simulink model "Warmup"  (R2012b)
settings: Solver=ode1  StartTime=0.0  StopTime=inf  FixedStep=0.001  RelTol=1e-3
PreLoadFcn:
  | prompt = {'Stimulation amplitude [mA]:','Number of pulses:'};
  | dlg_title = 'Warmup Settings';
  | def = {'50','20'};
  | answer = inputdlg(prompt,dlg_title,1,def);
  | amp = str2num(answer{1});
  | np = 1:str2num(answer{2});
  | clear prompt dlg_title def answer
undefined symbols (not defined in the file): HIL, LCconv
libraries: quarc_library x3, simulink x2, ScienceStimHasomed_Lib x1
settings Model: SimulationMode=external  ExtModeTrigDuration=5000000  Creator=LabUser  LastModifiedBy=LabUser
settings SolverCC: PositivePriorityOrder=on
settings DataIOCC: LimitDataPoints=off
settings DebuggingCC: SolverPrmCheckMsg=none
settings RTWCC: SystemTargetFile=quarc_win64.tlc  TemplateMakefile=quarc_default_tmf  Description=QUARC Win64 Target  ProcessScript=quarc_win64_make_rtw_hook
settings RTWCC: CustomLibrary=|
  | sciencemode.obj
  | serial_windows.obj
settings STFCustomTargetCC: TargetPreCompLibLocation=C:\PROGRA~3\QUARC\lib\2012b\win64\release  CodeReplacementLibrary=ANSI_C  GeneratePreprocessorConditionals=Disable all  CombineOutputUpdateFcns=on  GRTInterface=off  SystemTargetFile=quarc_win64.tlc
settings GRTTargetCC: TargetPreCompLibLocation=C:\PROGRA~3\QUARC\lib\2012b\win64\release  ParMdlRefBuildCompliant=off  CompOptLevelCompliant=off  ConcurrentExecutionCompliant=off  MatFileLogging=off  ExtMode=on  ExtModeMexFile=quarc_comm

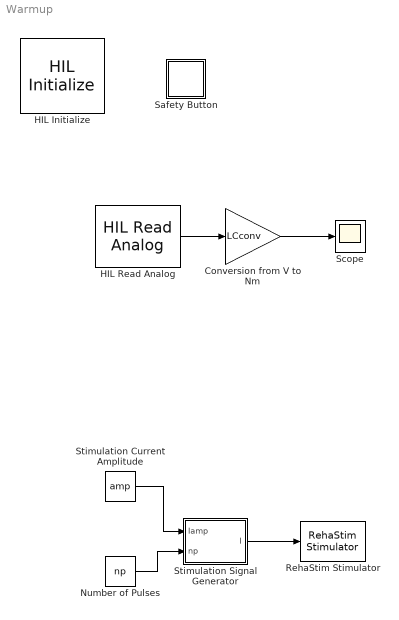
== system Warmup ==
  Conversion from V to Nm : Gain  Gain=LCconv
  HIL Initialize : quarc_library/Data Acquisition/Generic/Configuration/HIL Initialize  Priority=-99  object_name=HIL-1  board_type=qpid_e  board_number=0  board_options=enc0_dir=0;enc0_filter=1;enc0_a=1;enc0_b=1;enc0_z=0;enc0_reload=0;enc1_dir=0;enc1_filter=1;enc1_a=1;enc1_b=1;enc1_z=0;enc1_reload=0;enc2_dir=0;enc2_filter=1;enc2_a=1;enc2_b=1;enc2_z=0;enc2_reload=0;enc3_dir=0;enc3_filter=1;enc3_a=1;enc3_b=1;enc3_z=0;enc3_reload=0;enc4_dir=0;enc4_filter=1;enc4_a=1;enc4_b=1;enc4_z=0;enc4_reload=0;enc5_dir=0;enc5_filter=1;enc5_a=1;enc5_b=1;enc5_z=0;enc5_reload=0;enc6_dir=0;enc6_filter=1;enc6_a=1;enc6_b=1;enc6_z=0;enc6_reload=0;enc7_dir=0;enc7_filter=1;enc7_a=1;enc7_b=1;enc7_z=0;enc7_reload=0;ext_int_polarity=0;fuse_polarity=0;convert_polarity=0;watchdog_polarity=0;ext_int_watchdog=0;fuse_watchdog=0;trig1_watchdog=0;watchdog_to_trig1=0;watchdog_to_trig2=0;counter_to_trig0=0;trigger_adcs=0;latch_on_adc=0;pwm_immediate=0  exclusive=off  active=off  hardware_clocks=[0:16]  clock_modes=[]  initial_clock_frequencies=[]  set_clock_params_at_start=off  set_clock_params_at_switch_in=off  set_clock_frequencies_at_start=off  set_clock_frequencies_at_switch_in=off  analog_input_channels=[0:7]  analog_input_maximums=10  analog_input_minimums=-10  set_analog_input_params_at_start=off  set_analog_input_params_at_switch_in=off  analog_output_channels=[0:7]  analog_output_maximums=10  analog_output_minimums=-10  initial_analog_outputs=[0]  final_analog_outputs=[0]  watchdog_analog_outputs=0  set_analog_output_params_at_start=off  set_analog_output_params_at_switch_in=off  set_analog_outputs_at_start=on  set_analog_outputs_at_switch_in=off  set_analog_outputs_at_terminate=on  set_analog_outputs_at_switch_out=off  set_analog_outputs_on_watchdog=off  digital_input_channels=[]  digital_output_channels=[]  digital_output_configuration=[]  initial_digital_outputs=[1]  final_digital_outputs=[1]  watchdog_digital_outputs=[2]  set_digital_output_params_at_start=off  set_digital_output_params_at_switch_in=off  set_digital_outputs_at_start=on  set_digital_outputs_at_switch_in=off  set_digital_outputs_at_terminate=on  set_digital_outputs_at_switch_out=off  set_digital_outputs_on_watchdog=off  encoder_channels=[0:7]  quadrature=[4]  encoder_filter_frequency=40e6/1  initial_encoder_counts=[0]  set_encoder_params_at_start=off  set_encoder_params_at_switch_in=off  set_encoder_counts_at_start=off  set_encoder_counts_at_switch_in=off  pwm_channels=[0:7]  pwm_modes=0  pwm_frequency=40e6/4096  pwm_configuration=[0]  pwm_alignment=[0]  pwm_polarity=[1]  pwm_leading_deadband=[0]  pwm_trailing_deadband=[0]  initial_pwm_outputs=[0]  final_pwm_outputs=[0]  watchdog_pwm_outputs=[0]  set_pwm_params_at_start=on  set_pwm_params_at_switch_in=off  set_pwm_outputs_at_start=on  set_pwm_outputs_at_switch_in=off  set_pwm_outputs_at_terminate=on  set_pwm_outputs_at_switch_out=off  set_pwm_outputs_on_watchdog=off  other_output_channels=[]  initial_other_outputs=[]  final_other_outputs=[]  watchdog_other_outputs=[]  set_other_outputs_at_start=off  set_other_outputs_at_switch_in=off  set_other_outputs_at_terminate=off  set_other_outputs_at_switch_out=off  set_other_outputs_on_watchdog=off
  HIL Read Analog : quarc_library/Data Acquisition/Generic/Immediate I//O/HIL Read Analog  object_name=HIL-1  channels=0  sample_time=qc_get_step_size  active=on  vector_output=off
  Number of Pulses : Constant  Value=np
  RehaStim Stimulator : ScienceStimHasomed_Lib/RehaStim Stimulator  sFreq=1000  Freq=stimfreq  PWidth=PW
  Safety Button : Subsystem
  Scope : Scope
      settings: TimeRange=5  YMin=2.5  YMax=40  MaxDataPoints=500000
  Stimulation Current Amplitude : Constant  Value=amp
  Stimulation Signal Generator : Subsystem
  wires:
  HIL Read Analog/1 -> Conversion from V to Nm/1
  Conversion from V to Nm/1 -> Scope/1
  Stimulation Current Amplitude/1 -> Stimulation Signal Generator/1(Iamp)
  Stimulation Signal Generator/1(I) -> RehaStim Stimulator/1
  Number of Pulses/1 -> Stimulation Signal Generator/2(np)

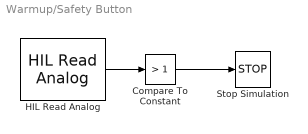
== system Warmup/Safety Button ==
  Compare To Constant : simulink/Logic and Bit Operations/Compare To Constant  relop=>  const=1  OutDataTypeStr=boolean
  HIL Read Analog : quarc_library/Data Acquisition/Generic/Immediate I//O/HIL Read Analog  object_name=HIL-1  channels=[7]  sample_time=qc_get_step_size  active=on  vector_output=off
  Stop Simulation : Stop
  wires:
  HIL Read Analog/1 -> Compare To Constant/1
  Compare To Constant/1 -> Stop Simulation/1

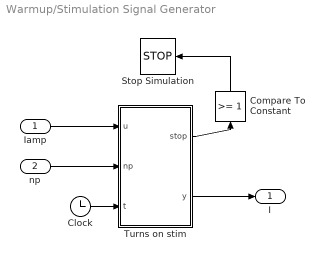
== system Warmup/Stimulation Signal Generator ==
  Iamp : Inport
  np : Inport  Port=2
  Clock : Clock
  Compare To Constant : simulink/Logic and Bit Operations/Compare To Constant  relop=>=  const=1  OutDataTypeStr=boolean
  Stop Simulation : Stop
  Turns on stim : MATLAB Function  TreatAsAtomicUnit=on
  I : Outport
  wires:
  Iamp/1 -> Turns on stim/1(u)
  Clock/1 -> Turns on stim/3(t)
  Turns on stim/2(y) -> I/1
  Turns on stim/1(stop) -> Compare To Constant/1
  Compare To Constant/1 -> Stop Simulation/1
  np/1 -> Turns on stim/2(np)

== matlab function Warmup/Stimulation Signal Generator/Turns on stim ==
  data: stop output; u input; np input; y output; t input
function [stop,y] = fcn(u,np,t)

%% Stimualtion Time Settings

% Time between warmup pulses [s]
dtw = 5;

% Note: The warmup and recovery pulses have a duration of 0.5s
dt = 0.5;

%% Stimulation Pulse Logic

% Total time for warmup
tw = max(np)*(dtw+dt);
% Warmup start time
twstart = 0;

if (t >= twstart) && (t <= twstart+tw)
    % This is the time when the warmup stimulation is applied.
    trel = t-twstart;
    
    if any((trel >= ((np)-1)*dt+(np)*dtw) + (trel <= (np)*(dtw+dt)) == 2)
        y = u;
    else
        y = 0;
    end
  
else
    % Otherwise do not output a stimulation.
    y = 0;
end


%% Simulation Stop Logic

if t < dtw+dt+tw
    stop = 0;
else
    stop = 1;
end
